simulink model "FBR_Buck_Sim"  (R2022b)
settings: Solver=VariableStepAuto  StartTime=0.0  StopTime=0.04  RelTol=1e-3
libraries: spsDiodeLib x7, spsACVoltageSourceLib x3, spsCurrentMeasurementLib x3, spsSeriesRLCBranchLib x2, spsVoltageMeasurementLib x2, spsDCVoltageSourceLib x1, spsIGBTLib x1, spsMeanLib x1, eePwmGenerator x1, sps_lib x1
settings Model: Creator=Mekatrona  LastModifiedBy=Mekatrona

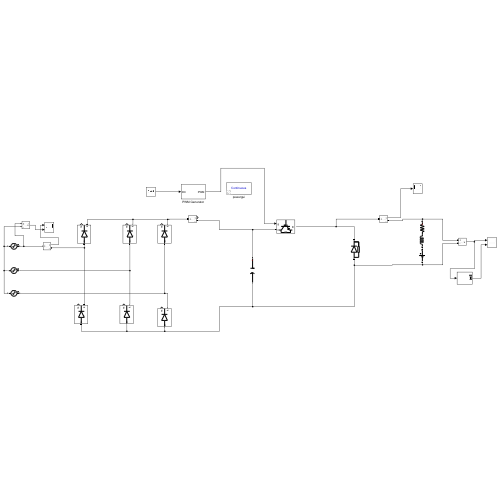
[thumbnail: Simulink's stored preview of the top-level diagram]
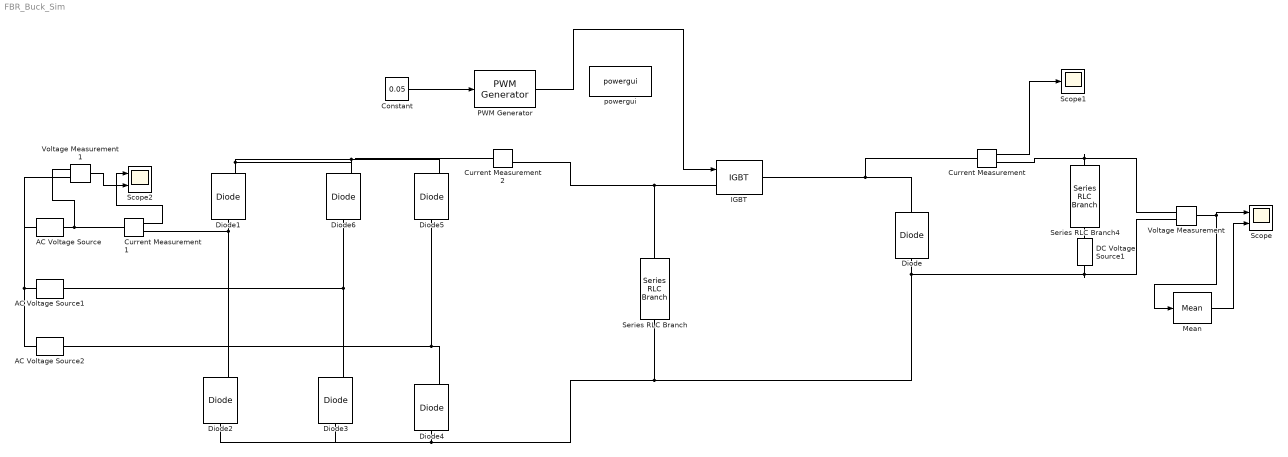
== system FBR_Buck_Sim ==
  AC Voltage Source : spsACVoltageSourceLib/AC Voltage Source  Amplitude=160  Phase=0  Frequency=50  SampleTime=0  Measurements=None  BusType=swing  Pref=10e3  Qref=0  Qmin=-inf  Qmax=+inf
  AC Voltage Source1 : spsACVoltageSourceLib/AC Voltage Source  Amplitude=160  Phase=120  Frequency=50  SampleTime=0  Measurements=None  BusType=swing  Pref=10e3  Qref=0  Qmin=-inf  Qmax=+inf
  AC Voltage Source2 : spsACVoltageSourceLib/AC Voltage Source  Amplitude=160  Phase=240  Frequency=50  SampleTime=0  Measurements=None  BusType=swing  Pref=10e3  Qref=0  Qmin=-inf  Qmax=+inf
  Constant : Constant  Value=0.05
  Current Measurement : spsCurrentMeasurementLib/Current Measurement  PhasorSimulation=off  OutputType=Complex  PSBequivalent=0
  Current Measurement1 : spsCurrentMeasurementLib/Current Measurement  PhasorSimulation=off  OutputType=Complex  PSBequivalent=0
  Current Measurement2 : spsCurrentMeasurementLib/Current Measurement  PhasorSimulation=off  OutputType=Complex  PSBequivalent=0
  DC Voltage Source1 : spsDCVoltageSourceLib/DC Voltage Source  Amplitude=0.05  Measurements=None
  Diode : spsDiodeLib/Diode  Ron=0.001  Lon=0  Vf=0.8  IC=0  UseSnubber=0  Rs=500  Cs=250e-9  Measurements=off
  Diode{1..6} (6 alike) : spsDiodeLib/Diode  Ron=0.001  Lon=0  Vf=0.8  IC=0  UseSnubber=0  Rs=0  Cs=0  Measurements=on
  IGBT : spsIGBTLib/IGBT  Ron=0.001  Lon=0  Vf=1  Tf=1e-6  Tt=2e-6  IC=0  Rs=1e5  Cs=inf  Measurements=off
  Mean : spsMeanLib/Mean  Freq=1000  Vinit=0  Ts=0
  PWM Generator : eePwmGenerator/PWM Generator  CarrCount=Up  Tper=1e-3  Tdelay=0  Ts=0
  Scope : Scope  NumInputPorts=2
  Scope1 : Scope
  Scope2 : Scope  NumInputPorts=2
  Series RLC Branch : spsSeriesRLCBranchLib/Series RLC Branch  LConnTagsString=__new0  RConnTagsString=__new0  BranchType=C  Resistance=1  Inductance=1e-3  SetiL0=off  InitialCurrent=0  Capacitance=470e-6  Setx0=off  InitialVoltage=0  Measurements=None
  Series RLC Branch4 : spsSeriesRLCBranchLib/Series RLC Branch  LConnTagsString=__new0  RConnTagsString=__new0  BranchType=RL  Resistance=0.8  Inductance=12.5e-3  SetiL0=off  InitialCurrent=0  Capacitance=1e-6  Setx0=off  InitialVoltage=0  Measurements=None
  Voltage Measurement : spsVoltageMeasurementLib/Voltage Measurement  PhasorSimulation=off  OutputType=Complex  PSBequivalent=0
  Voltage Measurement1 : spsVoltageMeasurementLib/Voltage Measurement  PhasorSimulation=off  OutputType=Complex  PSBequivalent=0
  powergui : sps_lib/powergui  Priority=1  SimulationMode=Continuous  SampleTime=50e-6  frequency=60  Iterations=50  frequencyindice=0  Pbase=100e6  ErrMax=1e-4  UnitsV=kV  UnitsW=MW  buscounter=0  FunctionMessages=off  echomessages=off  EnableUseOfTLC=off  CurrentSourceSwitches=off  DisableSnubberDevices=off  DisableRonSwitches=off  DisableVfSwitches=off  DisplayEquations=off  AutomaticDiscreteSolvers=off  SolverType=Tustin/Backward Euler (TBE)  Interpol=off  ExternalGateDelay=off  methode=off  Ts=100  x0status=blocks  SPID=on  SwTol=0  HookPort=off  NonlinearTolerance=1e-4  nMaxIteration=100  ContinueOnMaxIteration=off  RestoreLinks=warning  ResistiveCurrentMeasurement=off  Frange=[0:2:500]  Ylog=off  Xlog=on  ShowGrid=off  save=off  variable=ZData  structure=0  ZoomFFT=off  StartTime=0.0  cycles=1  DisplayStyle=1  fundamental=60  FreqAxis=off  MaxFrequency=1000  frequencyindicesteady=1  RmsSteady=1  display=off
  wires:
  PWM Generator/1 -> IGBT/1
  Constant/1 -> PWM Generator/1
  Voltage Measurement/1 -> Mean/1, Scope/1
  Mean/1 -> Scope/2
  Current Measurement/1 -> Scope1/1
  Voltage Measurement1/1 -> Scope2/2
  Current Measurement1/1 -> Scope2/1
  connections:
  Series RLC Branch4/LConn1 -- Current Measurement/RConn1 -- Voltage Measurement/LConn1
  Diode/RConn1 -- IGBT/RConn1 -- Current Measurement/LConn1
  DC Voltage Source1/RConn1 -- Series RLC Branch4/RConn1
  Voltage Measurement/LConn2 -- DC Voltage Source1/LConn1 -- Series RLC Branch/RConn1 -- Diode4/LConn1 -- Diode2/LConn1 -- Diode3/LConn1 -- Diode/LConn1
  Current Measurement2/RConn1 -- IGBT/LConn1 -- Series RLC Branch/LConn1
  Diode1/RConn1 -- Current Measurement2/LConn1 -- Diode5/RConn1 -- Diode6/RConn1
  AC Voltage Source1/LConn1 -- AC Voltage Source2/LConn1 -- AC Voltage Source/LConn1 -- Voltage Measurement1/LConn2
  Diode5/LConn1 -- AC Voltage Source2/RConn1 -- Diode4/RConn1
  Diode1/LConn1 -- Current Measurement1/RConn1 -- Diode2/RConn1
  AC Voltage Source/RConn1 -- Current Measurement1/LConn1 -- Voltage Measurement1/LConn1
  Diode6/LConn1 -- AC Voltage Source1/RConn1 -- Diode3/RConn1
